simulink model "radia_peec_coil_rlc_plant"  (R2026a)
settings: Solver=ode45  StopTime=0.012  MaxStep=1e-5  RelTol=1e-9  AbsTol=1e-11
PreLoadFcn:
  | R_ohm=0.02; L_H=8e-6; C_F=3.3e-3;
settings Model: Creator=Administrator  LastModifiedBy=Administrator

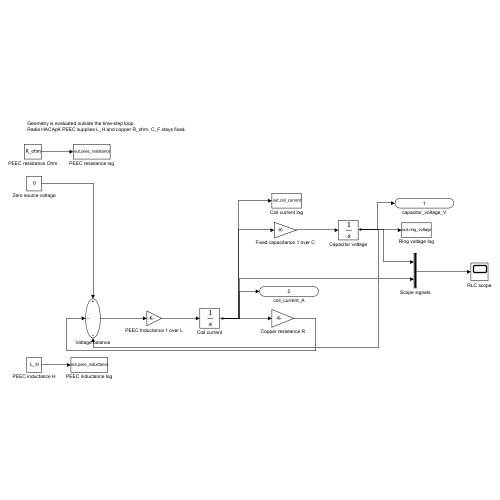
[thumbnail: Simulink's stored preview of the top-level diagram]
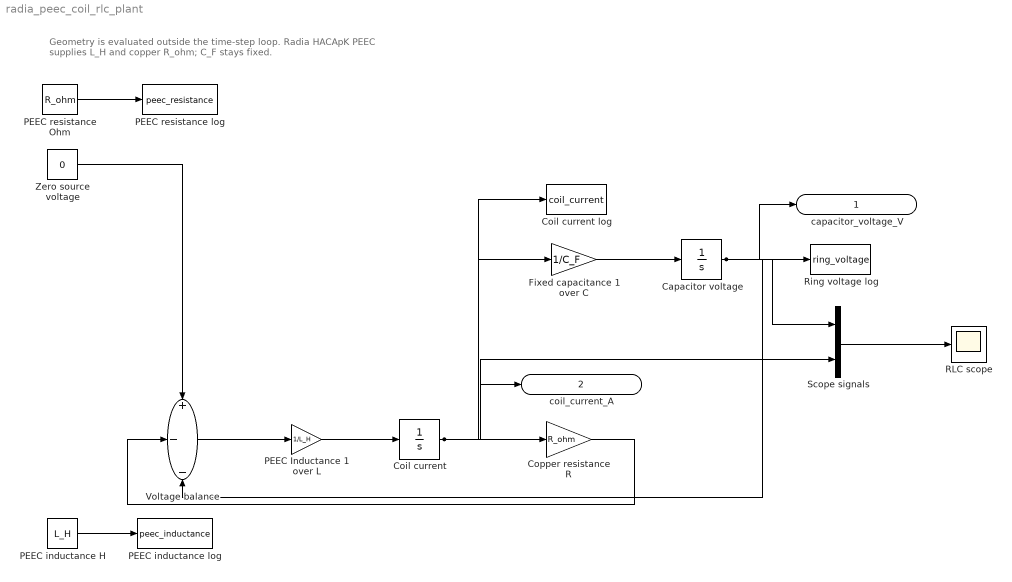
== system radia_peec_coil_rlc_plant ==
  note: Geometry is evaluated outside the time-step loop.
      | Radia HACApK PEEC supplies L_H and copper R_ohm; C_F stays fixed.
  Capacitor voltage : Integrator  InitialCondition=1
  Coil current : Integrator
  Coil current log : ToWorkspace  VariableName=coil_current  SaveFormat=Timeseries  SampleTime=-1
  Copper resistance R : Gain  Gain=R_ohm
  Fixed capacitance 1 over C : Gain  Gain=1/C_F
  PEEC Inductance 1 over L : Gain  Gain=1/L_H
  PEEC inductance H : Constant  Value=L_H
  PEEC inductance log : ToWorkspace  VariableName=peec_inductance  SaveFormat=Timeseries  SampleTime=-1
  PEEC resistance Ohm : Constant  Value=R_ohm
  PEEC resistance log : ToWorkspace  VariableName=peec_resistance  SaveFormat=Timeseries  SampleTime=-1
  RLC scope : Scope
  Ring voltage log : ToWorkspace  VariableName=ring_voltage  SaveFormat=Timeseries  SampleTime=-1
  Scope signals : Mux  Inputs=2
  Voltage balance : Sum  Inputs=+--
  Zero source voltage : Constant  Value=0
  capacitor_voltage_V : Outport
  coil_current_A : Outport  Port=2
  wires:
  PEEC resistance Ohm/1 -> PEEC resistance log/1
  Zero source voltage/1 -> Voltage balance/1
  PEEC inductance H/1 -> PEEC inductance log/1
  PEEC Inductance 1 over L/1 -> Coil current/1
  Voltage balance/1 -> PEEC Inductance 1 over L/1
  Coil current/1 -> Fixed capacitance 1 over C/1, Coil current log/1, coil_current_A/1, Copper resistance R/1, Scope signals/2
  Copper resistance R/1 -> Voltage balance/2
  Fixed capacitance 1 over C/1 -> Capacitor voltage/1
  Capacitor voltage/1 -> Ring voltage log/1, capacitor_voltage_V/1, Voltage balance/3, Scope signals/1
  Scope signals/1 -> RLC scope/1
